simulink model "Light_System_simulink"  (R2019b)
settings: Solver=VariableStepAuto  StartTime=0.0  StopTime=inf  RelTol=1e-3
libraries: simulink x5
settings Model: EnablePacing=on  Creator=Δημήτρης  LastModifiedBy=Εμμανουήλ
settings SolverCC: ZeroCrossAlgorithm=Adaptive  AlgebraicLoopSolver=LineSearch
settings DebuggingCC: IgnoredZcDiagnostic=none

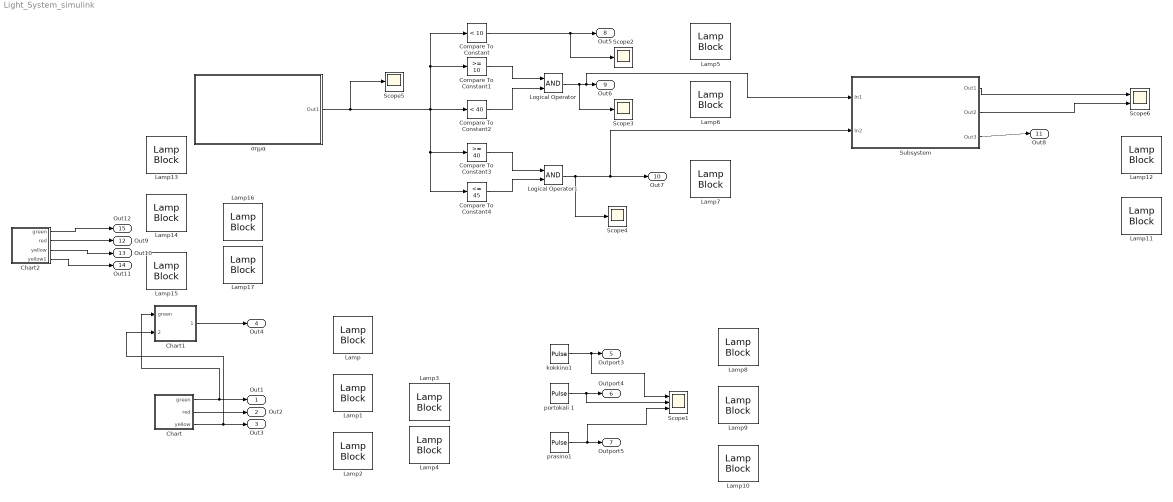
== system Light_System_simulink ==
  Chart : Stateflow chart  BlockKeywords=__PRM__SERIALIZED__DATA__:Stateflow Chart,Stateflow Diagram  TreatAsAtomicUnit=on
  Chart1 : Stateflow chart  BlockKeywords=__PRM__SERIALIZED__DATA__:Stateflow Chart,Stateflow Diagram  TreatAsAtomicUnit=on
  Chart2 : Stateflow chart  BlockKeywords=__PRM__SERIALIZED__DATA__:Stateflow Chart,Stateflow Diagram  TreatAsAtomicUnit=on
  Compare To Constant : simulink/Logic and Bit Operations/Compare To Constant  relop=<  const=10  OutDataTypeStr=boolean
  Compare To Constant1 : simulink/Logic and Bit Operations/Compare To Constant  relop=>=  const=10  OutDataTypeStr=boolean
  Compare To Constant2 : simulink/Logic and Bit Operations/Compare To Constant  relop=<  const=40  OutDataTypeStr=boolean
  Compare To Constant3 : simulink/Logic and Bit Operations/Compare To Constant  relop=>=  const=40  OutDataTypeStr=boolean
  Compare To Constant4 : simulink/Logic and Bit Operations/Compare To Constant  relop=<=  const=45  OutDataTypeStr=boolean
  Lamp{,1..17} (18 alike) : LampBlock
  Logical Operator : Logic  AllPortsSameDT=off  OutDataTypeStr=boolean
  Logical Operator1 : Logic  AllPortsSameDT=off  OutDataTypeStr=boolean
  Scope1 : Scope  NumInputPorts=3
  Scope{2..5} (4 alike) : Scope
  Scope6 : Scope  NumInputPorts=2
  Subsystem : Subsystem
  kokkino1 : DiscretePulseGenerator  PulseType=Time based  Period=45  PulseWidth=22.222222222
  portokali 1 : DiscretePulseGenerator  PulseType=Time based  Period=45  PulseWidth=11.11111111111  PhaseDelay=40
  prasino1 : DiscretePulseGenerator  PulseType=Time based  Period=45  PulseWidth=66.66666666666  PhaseDelay=10
  σημα : Subsystem
  Out1 : Outport
  Out2 : Outport  Port=2
  Out3 : Outport  Port=3
  Out4 : Outport  Port=4
  Outport3 : Outport  Port=5
  Outport4 : Outport  Port=6
  Outport5 : Outport  Port=7
  Out5 : Outport  Port=8
  Out6 : Outport  Port=9
  Out7 : Outport  Port=10
  Out8 : Outport  Port=11
  Out9 : Outport  Port=12
  Out10 : Outport  Port=13
  Out11 : Outport  Port=14
  Out12 : Outport  Port=15
  wires:
  Chart/2(red) -> Out2/1
  Chart/3(yellow) -> Chart1/2(yellow), Out3/1
  Chart/1(green) -> Chart1/1(green), Out1/1
  Chart1/1(yellow1) -> Out4/1
  prasino1/1 -> Outport5/1, Scope1/3
  portokali 1/1 -> Outport4/1, Scope1/2
  kokkino1/1 -> Outport3/1, Scope1/1
  Compare To Constant/1 -> Out5/1, Scope2/1
  Compare To Constant1/1 -> Logical Operator/1
  Compare To Constant2/1 -> Logical Operator/2
  Compare To Constant3/1 -> Logical Operator1/1
  Compare To Constant4/1 -> Logical Operator1/2
  Logical Operator1/1 -> Scope4/1, Subsystem/2(In2), Out7/1
  σημα/1(Out1) -> Scope5/1, Compare To Constant4/1, Compare To Constant3/1, Compare To Constant2/1, Compare To Constant/1, Compare To Constant1/1
  Logical Operator/1 -> Subsystem/1(In1), Out6/1, Scope3/1
  Subsystem/1(Out1) -> Scope6/1
  Subsystem/2(Out2) -> Scope6/2
  Subsystem/3(Out3) -> Out8/1
  Chart2/1(green) -> Out12/1
  Chart2/2(red) -> Out9/1
  Chart2/3(yellow) -> Out10/1
  Chart2/4(yellow1) -> Out11/1

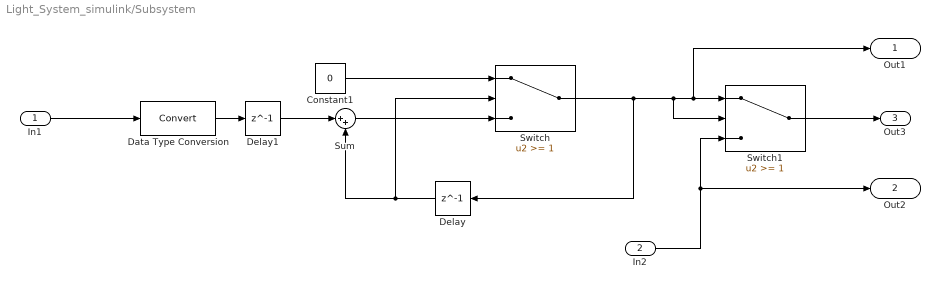
== system Light_System_simulink/Subsystem ==
  In1 : Inport
  In2 : Inport  Port=2
  Constant1 : Constant  Value=0
  Data Type Conversion : DataTypeConversion
  Delay : Delay  DelayLength=1  InitialCondition=0  SampleTime=1
  Delay1 : Delay  DelayLength=1  InitialCondition=0  SampleTime=1
  Sum : Sum  Inputs=|++
  Switch : Switch  Threshold=1
  Switch1 : Switch  Threshold=1
  Out1 : Outport
  Out2 : Outport  Port=2
  Out3 : Outport  Port=3
  wires:
  Data Type Conversion/1 -> Delay1/1
  Constant1/1 -> Switch/1
  Delay1/1 -> Sum/1
  In1/1 -> Data Type Conversion/1
  Switch1/1 -> Out3/1
  Switch/1 -> Out1/1, Switch1/1, Switch1/2, Delay/1
  In2/1 -> Switch1/3, Out2/1
  Sum/1 -> Switch/3
  Delay/1 -> Sum/2, Switch/2

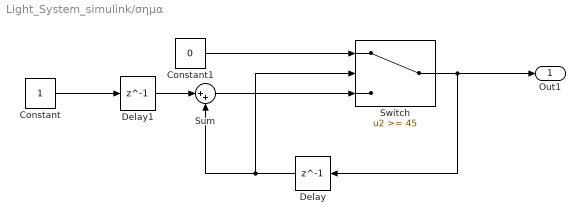
== system Light_System_simulink/σημα ==
  Constant : Constant
  Constant1 : Constant  Value=0
  Delay : Delay  DelayLength=1  InitialCondition=0  SampleTime=1
  Delay1 : Delay  DelayLength=1  InitialCondition=0  SampleTime=1
  Sum : Sum  Inputs=|++
  Switch : Switch  Threshold=45
  Out1 : Outport
  wires:
  Delay/1 -> Sum/2, Switch/2
  Sum/1 -> Switch/3
  Delay1/1 -> Sum/1
  Constant1/1 -> Switch/1
  Constant/1 -> Delay1/1
  Switch/1 -> Delay/1, Out1/1

== stateflow chart Light_System_simulink/Chart1 ==
  state yellow1
    yellow1 = 0;
  state yellow2
    yellow1 = 1;
  (default) -> yellow1
  yellow1 -> yellow2 [order 1] : [green==1]{after(3,sec)}
  yellow1 -> yellow2 [order 2] : [yellow==1]
  yellow2 -> yellow1 [order 2] : [yellow==0]
  yellow2 -> yellow1 [order 1] : [green==1]{after(3,sec)}
  data: green input; yellow1 output; yellow input

== stateflow chart Light_System_simulink/Chart2 ==
  state stop
    entry:
    red = 1;
    yellow = 0;
    green = 0;
  state start
    entry:
    red = 0;
    yellow = 0;
    green = 1;
  state preparetostop
    entry:
    red = 0;
    yellow = 1;
    green = 0;
  state Yellow1
    state yello_off
      entry:yellow1=0;
    state yello_on
      entry:yellow1=1;
    yello_off -> yello_on : after(1,sec)[green==1]
    (default) -> yello_off
    yello_on -> yello_off : after(1,sec)[green==1]
  (default) -> stop
  stop -> start : after(15,sec)
  start -> Yellow1 : [green==1]
  preparetostop -> stop : after(5,sec){yellow1=0}
  Yellow1 -> preparetostop : after(40,sec)
  data: green output; red output; yellow output; yellow1 output

== stateflow chart Light_System_simulink/Chart ==
  state stop
    entry:
    red = 1;
    yellow = 0;
    green = 0;
  state start1
    entry:
    red = 0;
    yellow = 0;
    green = 1;
  state preparetostop
    entry:
    red = 0;
    yellow = 1;
    green = 0;
  (default) -> stop
  stop -> start1 : after(10,sec)
  preparetostop -> stop : after(5,sec)
  start1 -> preparetostop : after(30,sec)
  data: green output; red output; yellow output
